simulink model "PassStCshnFldCtrl"  (R2018b)
settings: Solver=FixedStepDiscrete  StartTime=0.0  StopTime=10.0  RelTol=1e-3
undefined symbols (not defined in the file or in its folder): KeSMSuMdMotFinshdTm_Val, KeSMSuMdRetryTm1_Val, KeSMSuModeReqDurgTm_Val
libraries: StCtrlLib x1
settings Model: ModifiedHistory=2024.6.26 557模式流程V1.6  Creator=sn2xws  LastModifiedBy=sn2xws
settings DataIOCC: SaveFormat=StructureWithTime
settings OptimizationCC: DefaultParameterBehavior=Inlined  EnhancedBackFolding=on  PassReuseOutputArgsAs=Individual arguments  ZeroExternalMemoryAtStartup=off  ZeroInternalMemoryAtStartup=off  OptimizeBlockOrder=speed  DifferentSizesBufferReuse=on  OptimizationCustomize=off
settings DebuggingCC: ParameterTunabilityLossMsg=error
settings SFSimCC: MATLABDynamicMemAlloc=off
settings RTWCC: SystemTargetFile=autosar.tlc  GenCodeOnly=on  TemplateMakefile=ert_default_tmf  Description=AUTOSAR  GenerateReport=on  IncludeHyperlinkInReport=on  LaunchReport=on  GenerateTraceInfo=on  GenerateTraceReport=on  GenerateTraceReportSl=on  GenerateTraceReportSf=on  GenerateTraceReportEml=on
settings CodeAppCC: ForceParamTrailComments=on  IgnoreCustomStorageClasses=off  OperatorAnnotations=on  SimulinkDataObjDesc=on  SFDataObjDesc=on  InsertBlockDesc=on
settings STFCustomTargetCC: TargetLangStandard=C99 (ISO)  MultiwordLength=256  ParMdlRefBuildCompliant=on  CompOptLevelCompliant=on  IncludeMdlTerminateFcn=off  CombineOutputUpdateFcns=on  SuppressErrorStatus=on  ERTCustomFileBanners=on  SupportNonFinite=off  SupportComplex=off  SupportContinuousTime=off  SupportNonInlinedSFcns=off  RemoveResetFunc=on  MATLABClassNameForMDSCustomization=Simulink.SoftwareTarget.ERTCustomization  AutosarCompliant=on  UseToolchainInfoCompliant=on  LookupTableObjectStructAxisOrder=2,1,3,4,...  LUTObjectStructOrderEvenSpacing=Size,Table,Breakpoints  SystemTargetFile=autosar.tlc
settings ERTTargetCC: TargetLangStandard=C99 (ISO)  ConcurrentExecutionCompliant=off  IncludeMdlTerminateFcn=off  SuppressErrorStatus=on  SupportNonFinite=off  SupportComplex=off  ModelStepFunctionPrototypeControlCompliant=off  CPPClassGenCompliant=off  AutosarCompliant=on  LookupTableObjectStructAxisOrder=2,1,3,4,...  LUTObjectStructOrderEvenSpacing=Size,Table,Breakpoints  InlinedParameterPlacement=NonHierarchical  ERTCustomFileTemplate=example_file_process.tlc  ERTFilePackagingFormat=Compact

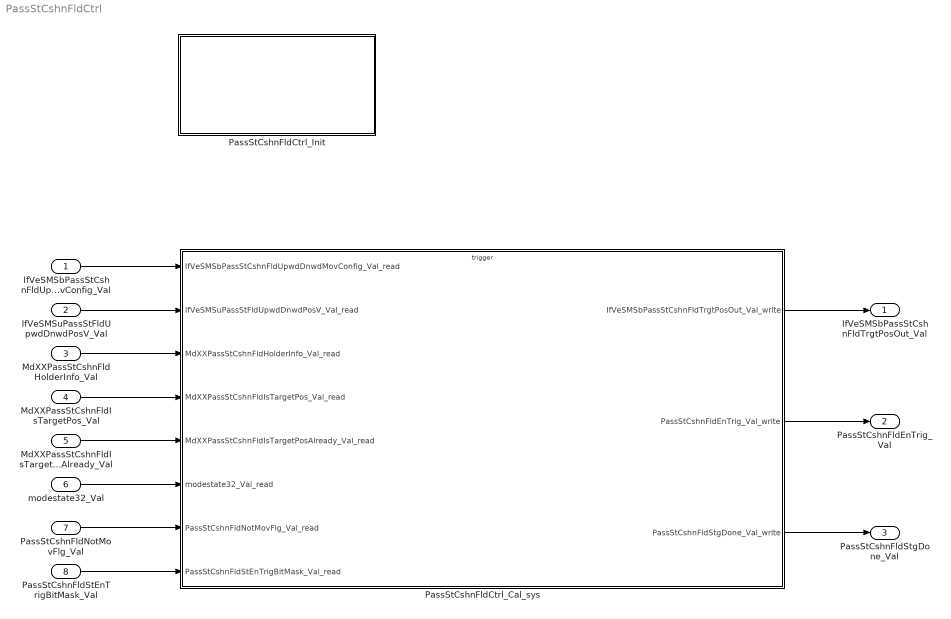
== system PassStCshnFldCtrl ==
  IfVeSMSbPassStCshnFldUpwdDnwdMovConfig_Val : Inport  OutDataTypeStr=boolean  PortDimensions=1
  IfVeSMSuPassStFldUpwdDnwdPosV_Val : Inport  Port=2  OutDataTypeStr=boolean  PortDimensions=1
  MdXXPassStCshnFldHolderInfo_Val : Inport  Port=3  OutDataTypeStr=uint32  PortDimensions=1
  MdXXPassStCshnFldIsTargetPos_Val : Inport  Port=4  OutDataTypeStr=uint32  PortDimensions=1
  MdXXPassStCshnFldIsTargetPosAlready_Val : Inport  Port=5  OutDataTypeStr=uint32  PortDimensions=1
  modestate32_Val : Inport  Port=6  OutDataTypeStr=uint32  PortDimensions=1
  PassStCshnFldNotMovFlg_Val : Inport  Port=7  OutDataTypeStr=boolean  PortDimensions=1
  PassStCshnFldStEnTrigBitMask_Val : Inport  Port=8  OutDataTypeStr=uint32  PortDimensions=1
  PassStCshnFldCtrl_Cal_sys : Subsystem
  PassStCshnFldCtrl_Init : Subsystem
  IfVeSMSbPassStCshnFldTrgtPosOut_Val : Outport  OutDataTypeStr=boolean  PortDimensions=1
  PassStCshnFldEnTrig_Val : Outport  Port=2  OutDataTypeStr=boolean  PortDimensions=1
  PassStCshnFldStgDone_Val : Outport  Port=3  OutDataTypeStr=boolean  PortDimensions=1
  wires:
  IfVeSMSbPassStCshnFldUpwdDnwdMovConfig_Val/1 -> PassStCshnFldCtrl_Cal_sys/1(IfVeSMSbPassStCshnFldUpwdDnwdMovConfig_Val_read)
  IfVeSMSuPassStFldUpwdDnwdPosV_Val/1 -> PassStCshnFldCtrl_Cal_sys/2(IfVeSMSuPassStFldUpwdDnwdPosV_Val_read)
  MdXXPassStCshnFldHolderInfo_Val/1 -> PassStCshnFldCtrl_Cal_sys/3(MdXXPassStCshnFldHolderInfo_Val_read)
  MdXXPassStCshnFldIsTargetPos_Val/1 -> PassStCshnFldCtrl_Cal_sys/4(MdXXPassStCshnFldIsTargetPos_Val_read)
  MdXXPassStCshnFldIsTargetPosAlready_Val/1 -> PassStCshnFldCtrl_Cal_sys/5(MdXXPassStCshnFldIsTargetPosAlready_Val_read)
  modestate32_Val/1 -> PassStCshnFldCtrl_Cal_sys/6(modestate32_Val_read)
  PassStCshnFldNotMovFlg_Val/1 -> PassStCshnFldCtrl_Cal_sys/7(PassStCshnFldNotMovFlg_Val_read)
  PassStCshnFldStEnTrigBitMask_Val/1 -> PassStCshnFldCtrl_Cal_sys/8(PassStCshnFldStEnTrigBitMask_Val_read)
  PassStCshnFldCtrl_Cal_sys/1(IfVeSMSbPassStCshnFldTrgtPosOut_Val_write) -> IfVeSMSbPassStCshnFldTrgtPosOut_Val/1
  PassStCshnFldCtrl_Cal_sys/2(PassStCshnFldEnTrig_Val_write) -> PassStCshnFldEnTrig_Val/1
  PassStCshnFldCtrl_Cal_sys/3(PassStCshnFldStgDone_Val_write) -> PassStCshnFldStgDone_Val/1

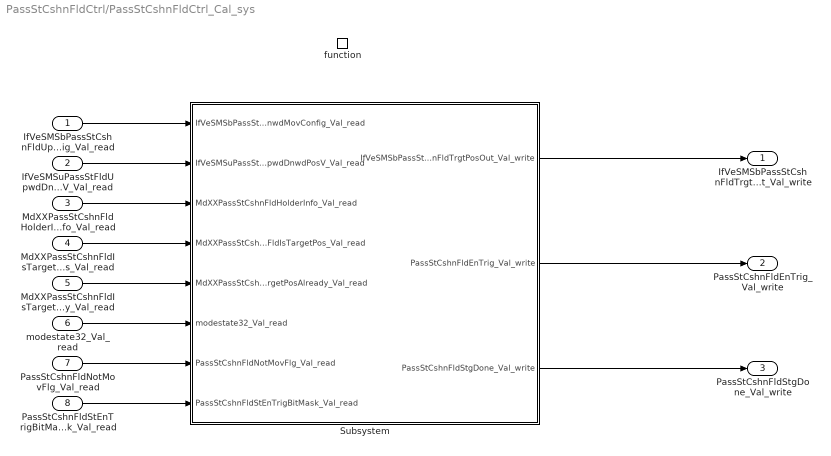
== system PassStCshnFldCtrl/PassStCshnFldCtrl_Cal_sys ==
  IfVeSMSbPassStCshnFldUpwdDnwdMovConfig_Val_read : Inport
  IfVeSMSuPassStFldUpwdDnwdPosV_Val_read : Inport  Port=2
  MdXXPassStCshnFldHolderInfo_Val_read : Inport  Port=3
  MdXXPassStCshnFldIsTargetPos_Val_read : Inport  Port=4
  MdXXPassStCshnFldIsTargetPosAlready_Val_read : Inport  Port=5
  modestate32_Val_read : Inport  Port=6
  PassStCshnFldNotMovFlg_Val_read : Inport  Port=7
  PassStCshnFldStEnTrigBitMask_Val_read : Inport  Port=8
  function : TriggerPort  TriggerType=function-call  IsSimulinkFunction=on  FunctionName=PassStCshnFldCtrl_Cal  VariantControl=(inherit)
  Subsystem : Subsystem
  IfVeSMSbPassStCshnFldTrgtPosOut_Val_write : Outport
      settings: EnsureOutportIsVirtual=on
  PassStCshnFldEnTrig_Val_write : Outport  Port=2
      settings: EnsureOutportIsVirtual=on
  PassStCshnFldStgDone_Val_write : Outport  Port=3
      settings: EnsureOutportIsVirtual=on
  wires:
  IfVeSMSbPassStCshnFldUpwdDnwdMovConfig_Val_read/1 -> Subsystem/1(IfVeSMSbPassStCshnFldUpwdDnwdMovConfig_Val_read)
  IfVeSMSuPassStFldUpwdDnwdPosV_Val_read/1 -> Subsystem/2(IfVeSMSuPassStFldUpwdDnwdPosV_Val_read)
  MdXXPassStCshnFldHolderInfo_Val_read/1 -> Subsystem/3(MdXXPassStCshnFldHolderInfo_Val_read)
  MdXXPassStCshnFldIsTargetPos_Val_read/1 -> Subsystem/4(MdXXPassStCshnFldIsTargetPos_Val_read)
  MdXXPassStCshnFldIsTargetPosAlready_Val_read/1 -> Subsystem/5(MdXXPassStCshnFldIsTargetPosAlready_Val_read)
  modestate32_Val_read/1 -> Subsystem/6(modestate32_Val_read)
  PassStCshnFldNotMovFlg_Val_read/1 -> Subsystem/7(PassStCshnFldNotMovFlg_Val_read)
  PassStCshnFldStEnTrigBitMask_Val_read/1 -> Subsystem/8(PassStCshnFldStEnTrigBitMask_Val_read)
  Subsystem/1(IfVeSMSbPassStCshnFldTrgtPosOut_Val_write) -> IfVeSMSbPassStCshnFldTrgtPosOut_Val_write/1
  Subsystem/2(PassStCshnFldEnTrig_Val_write) -> PassStCshnFldEnTrig_Val_write/1
  Subsystem/3(PassStCshnFldStgDone_Val_write) -> PassStCshnFldStgDone_Val_write/1

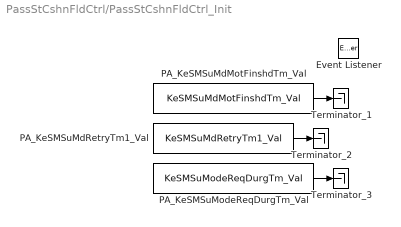
== system PassStCshnFldCtrl/PassStCshnFldCtrl_Init ==
  Event Listener : EventListener  EventName=reset
  PA_KeSMSuMdMotFinshdTm_Val : Constant  Value=KeSMSuMdMotFinshdTm_Val
  PA_KeSMSuMdRetryTm1_Val : Constant  Value=KeSMSuMdRetryTm1_Val
  PA_KeSMSuModeReqDurgTm_Val : Constant  Value=KeSMSuModeReqDurgTm_Val
  Terminator_1 : Terminator
  Terminator_2 : Terminator
  Terminator_3 : Terminator
  wires:
  PA_KeSMSuMdMotFinshdTm_Val/1 -> Terminator_1/1
  PA_KeSMSuMdRetryTm1_Val/1 -> Terminator_2/1
  PA_KeSMSuModeReqDurgTm_Val/1 -> Terminator_3/1

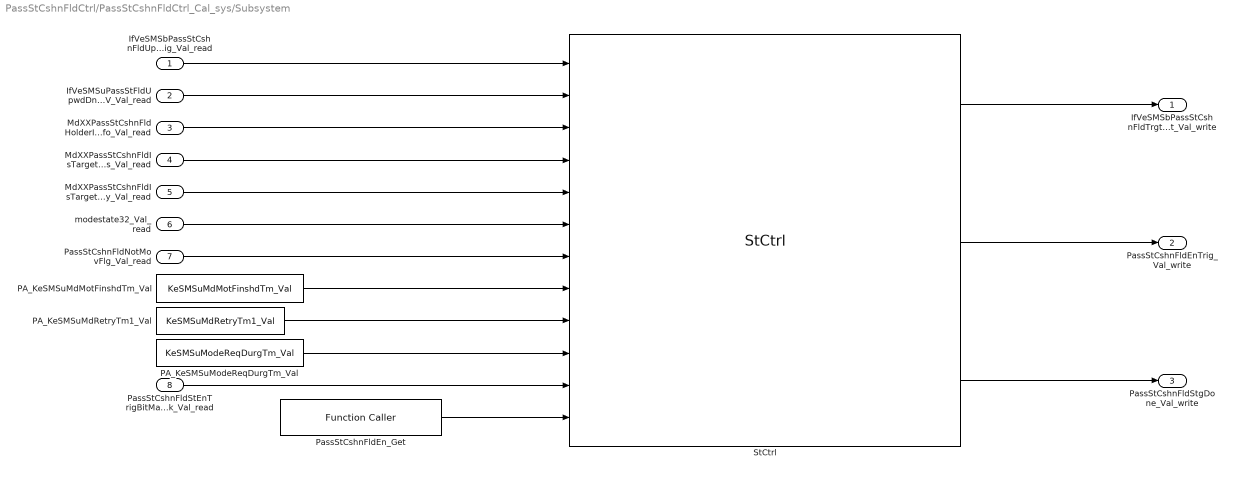
== system PassStCshnFldCtrl/PassStCshnFldCtrl_Cal_sys/Subsystem ==
  IfVeSMSbPassStCshnFldUpwdDnwdMovConfig_Val_read : Inport
  IfVeSMSuPassStFldUpwdDnwdPosV_Val_read : Inport  Port=2
  MdXXPassStCshnFldHolderInfo_Val_read : Inport  Port=3
  MdXXPassStCshnFldIsTargetPos_Val_read : Inport  Port=4
  MdXXPassStCshnFldIsTargetPosAlready_Val_read : Inport  Port=5
  modestate32_Val_read : Inport  Port=6
  PassStCshnFldNotMovFlg_Val_read : Inport  Port=7
  PassStCshnFldStEnTrigBitMask_Val_read : Inport  Port=8
  PA_KeSMSuMdMotFinshdTm_Val : Constant  Value=KeSMSuMdMotFinshdTm_Val
  PA_KeSMSuMdRetryTm1_Val : Constant  Value=KeSMSuMdRetryTm1_Val
  PA_KeSMSuModeReqDurgTm_Val : Constant  Value=KeSMSuModeReqDurgTm_Val
  PassStCshnFldEn_Get : FunctionCaller  FunctionPrototype=data = PassStCshnFldEn_Get()  OutputArgumentSpecifications=uint32(1)
  StCtrl : StCtrlLib/StCtrl  SystemSampleTime=-1
  IfVeSMSbPassStCshnFldTrgtPosOut_Val_write : Outport
      settings: EnsureOutportIsVirtual=on
  PassStCshnFldEnTrig_Val_write : Outport  Port=2
      settings: EnsureOutportIsVirtual=on
  PassStCshnFldStgDone_Val_write : Outport  Port=3
      settings: EnsureOutportIsVirtual=on
  wires:
  PassStCshnFldEn_Get/1 -> StCtrl/12
  StCtrl/1 -> IfVeSMSbPassStCshnFldTrgtPosOut_Val_write/1
  StCtrl/2 -> PassStCshnFldEnTrig_Val_write/1
  StCtrl/3 -> PassStCshnFldStgDone_Val_write/1
  IfVeSMSbPassStCshnFldUpwdDnwdMovConfig_Val_read/1 -> StCtrl/1
  IfVeSMSuPassStFldUpwdDnwdPosV_Val_read/1 -> StCtrl/2
  MdXXPassStCshnFldHolderInfo_Val_read/1 -> StCtrl/3
  MdXXPassStCshnFldIsTargetPos_Val_read/1 -> StCtrl/4
  MdXXPassStCshnFldIsTargetPosAlready_Val_read/1 -> StCtrl/5
  modestate32_Val_read/1 -> StCtrl/6
  PassStCshnFldNotMovFlg_Val_read/1 -> StCtrl/7
  PA_KeSMSuMdMotFinshdTm_Val/1 -> StCtrl/8
  PA_KeSMSuMdRetryTm1_Val/1 -> StCtrl/9
  PA_KeSMSuModeReqDurgTm_Val/1 -> StCtrl/10
  PassStCshnFldStEnTrigBitMask_Val_read/1 -> StCtrl/11
